simulink model "Sim8_1"  (R2023b)
settings: Solver=VariableStepAuto  StartTime=0.0  StopTime=10  FixedStep=0.001  RelTol=1e-3
InitFcn:
  | Parameters201201
values from neighbouring files (symbols this model uses):
  b0 = 0.6    [Parameters201201.m]
  N = 2    [Parameters201201.m]
  Wc = 10    [Parameters201201.m]
  Wo = 30    [Parameters201201.m]
  z0 = [0 0 0]    [Parameters201201.m]
settings Model: Creator=unive  LastModifiedBy=LG
settings SolverCC: AlgebraicLoopSolver=TrustRegion
settings DataIOCC: ReturnWorkspaceOutputs=off
settings DebuggingCC: AlgebraicLoopMsg=none  UnconnectedInputMsg=warning  UnconnectedOutputMsg=warning  UnconnectedLineMsg=warning  ArithmeticOperatorsInVariantConditions=warning
settings ModelReferenceCC: EnableRefExpFcnMdlSchedulingChecks=on
settings SFSimCC: SimUseLocalCustomCode=off  CustomCodeUndefinedFunction=UseInterfaceOnly
settings RTWCC: RTWUseLocalCustomCode=off
settings CodeAppCC: StateflowObjectComments=on

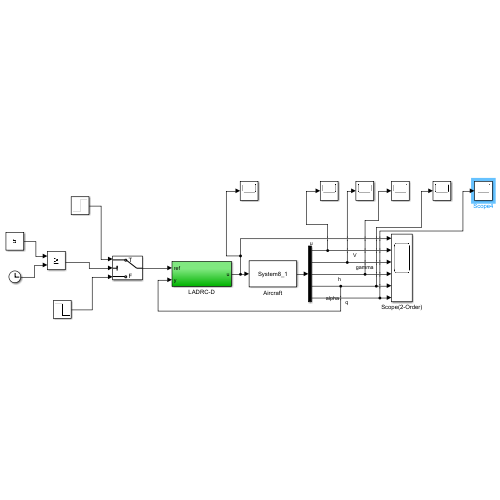
[thumbnail: Simulink's stored preview of the top-level diagram]
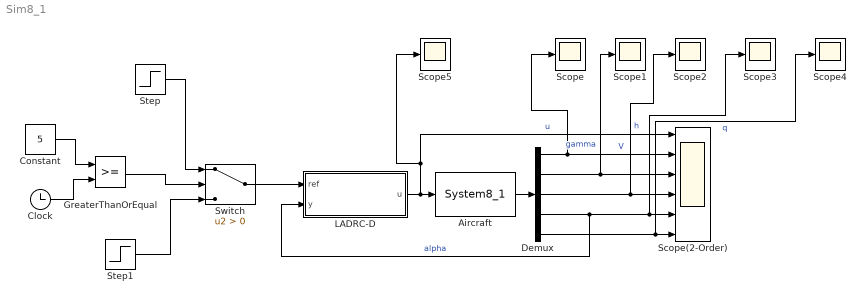
== system Sim8_1 ==
  Aircraft : S-Function  FunctionName=System8_1  Parameters=pa  SFunctionDeploymentMode=off  EnableBusSupport=off
  Clock : Clock
  Constant : Constant  Value=5
  Demux : Demux  Outputs=5
  GreaterThanOrEqual : RelationalOperator  OutDataTypeStr=boolean  RndMeth=Simplest  InputSameDT=off
  "LADRC-D " : Subsystem
  Scope{,1..5} (6 alike) : Scope
  Scope(2-Order) : Scope  NumInputPorts=6
  Step : Step  Time=0  After=0.1  SampleTime=0
  Step1 : Step  Time=0  After=-0.1  SampleTime=0
  Switch : Switch  Criteria=u2 > Threshold  SaturateOnIntegerOverflow=off  InputSameDT=off
  wires:
  "LADRC-D "/1(u) -> Scope5/1, Scope(2-Order)/1, Aircraft/1  "u"
  Aircraft/1 -> Demux/1
  Demux/1 -> Scope/1, Scope(2-Order)/2  "V"
  Demux/2 -> Scope1/1, Scope(2-Order)/3  "gamma"
  Demux/3 -> Scope2/1, Scope(2-Order)/4  "h"
  Demux/4 -> "LADRC-D "/2(y), Scope3/1, Scope(2-Order)/5  "alpha"
  Demux/5 -> Scope4/1, Scope(2-Order)/6  "q"
  Switch/1 -> "LADRC-D "/1(ref)
  Constant/1 -> GreaterThanOrEqual/1
  Clock/1 -> GreaterThanOrEqual/2
  GreaterThanOrEqual/1 -> Switch/2
  Step/1 -> Switch/1
  Step1/1 -> Switch/3

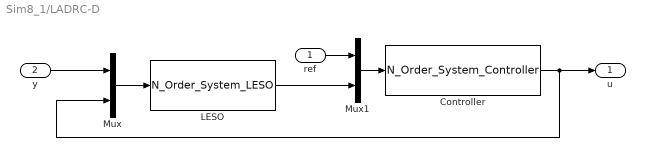
== system Sim8_1/LADRC-D  ==
  ref : Inport
  y : Inport  Port=2
  Controller : S-Function  FunctionName=N_Order_System_Controller  Parameters=N,Wc,b0  SFunctionDeploymentMode=off  EnableBusSupport=off
  LESO : S-Function  FunctionName=N_Order_System_LESO  Parameters=N,Wo,b0,z0  SFunctionDeploymentMode=off  EnableBusSupport=off
  Mux : Mux  Inputs=2
  Mux1 : Mux  Inputs=2
  u : Outport
  wires:
  y/1 -> Mux/1
  LESO/1 -> Mux1/2
  ref/1 -> Mux1/1
  Mux1/1 -> Controller/1
  Controller/1 -> Mux/2, u/1
  Mux/1 -> LESO/1
